simulink model "Laboratorio_5_SC2_Simulink_P3"  (R2019a)
settings: Solver=VariableStepAuto  StartTime=0.0  StopTime=1.5  RelTol=1e-3
values from neighbouring files (symbols this model uses):
  A_p3 = double(A_p3)    [Laboratorio_5_SC2.m]
  B_p3 = double(B_p3)    [Laboratorio_5_SC2.m]
  C1 = [1 0 0 0 ... (first row only)    [Laboratorio_5_SC2.m]
  C2 = eye(4)    [Laboratorio_5_SC2.m]
  D1 = [0; 0]    [Laboratorio_5_SC2.m]
  D2 = [0; 0; 0; 0]    [Laboratorio_5_SC2.m]
  F = 500e3    (= 500000)    [Laboratorio_5_SC2.m]
  fs_new = 20000    [Laboratorio_5_SC2.m]
  fv = 15020    [Laboratorio_5_SC2.m]
  init_con = [0; 1; 0; 0]    [Laboratorio_5_SC2.m]
libraries: fl_lib x13, nesl_utility x6
settings Model: Creator=Hector  LastModifiedBy=Hector

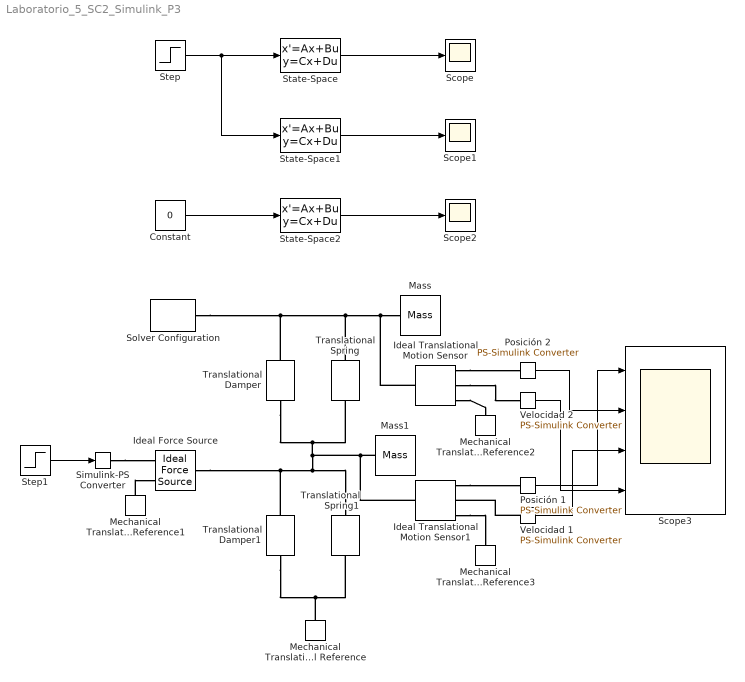
== system Laboratorio_5_SC2_Simulink_P3 ==
  Constant : Constant  Value=0
  Ideal Force Source : fl_lib/Mechanical/Mechanical Sources/Ideal Force Source
  Ideal Translational Motion Sensor : fl_lib/Mechanical/Mechanical Sensors/Ideal Translational Motion Sensor  offset=0 m
  Ideal Translational Motion Sensor1 : fl_lib/Mechanical/Mechanical Sensors/Ideal Translational Motion Sensor  offset=0 m
  Mass : fl_lib/Mechanical/Translational Elements/Mass  mass=M2 kg  v_specify=off  v_priority=High  v=0 m/s  v_nominal_specify=off  v_nominal_unit=m/s  v_nominal_value=1  f_specify=off  f_priority=None  f=0 N  f_nominal_specify=off  f_nominal_unit=N  f_nominal_value=1
  Mass1 : fl_lib/Mechanical/Translational Elements/Mass  mass=M1 kg  v_specify=off  v_priority=High  v=0 m/s  v_nominal_specify=off  v_nominal_unit=m/s  v_nominal_value=1  f_specify=off  f_priority=None  f=0 N  f_nominal_specify=off  f_nominal_unit=N  f_nominal_value=1
  Mechanical Translational Reference{,1..3} (4 alike) : fl_lib/Mechanical/Translational Elements/Mechanical Translational Reference
  Posición 1 : nesl_utility/PS-Simulink Converter  PhysicalDomain=network_engine_domain  SubClassName=ps_output  LeftPortType=input  RightPortType=output  PseudoPeriodic=off  Frequencies=[]  Unit=1  AffineConversion=off
  Posición 2 : nesl_utility/PS-Simulink Converter  PhysicalDomain=network_engine_domain  SubClassName=ps_output  LeftPortType=input  RightPortType=output  PseudoPeriodic=off  Frequencies=[]  Unit=1  AffineConversion=off
  Scope : Scope
  Scope1 : Scope
  Scope2 : Scope
  Scope3 : Scope  NumInputPorts=4
  Simulink-PS Converter : nesl_utility/Simulink-PS Converter  PhysicalDomain=network_engine_domain  SubClassName=ps_input  LeftPortType=input  RightPortType=output  PseudoPeriodic=off  Frequencies=[]  NoiseDistribution=none  NoiseParameters=[]  Unit=1  AffineConversion=off  FilteringAndDerivatives=provide  SimscapeFilterOrder=1  InputFilterTimeConstant=0.001  UdotUserProvided=0
  Solver Configuration : nesl_utility/Solver Configuration  PhysicalDomain=network_engine_domain  SubClassName=solver  LeftPortType=input  RightPortType=generic  Tones=[]  Harmonics=[]  SimulateNoise=off  Profile=off  UseLocalSampling=off  EnableSwitchedLinearOptims=on  FrequencyDomain=off  UseCCode=off  RelTol=0.001  AbsTol=1e-06  MinStep=1e-09  ToWorkspace=off  RevertToSquareIcSolve=off  NumHomotopyIterations=100  PhasorMode=off  PhasorModeNumHarmonics=1  DoDC=off  ResidualTolerance=1e-09  UseLocalSolver=off  LocalSolverChoice=NE_BACKWARD_EULER_ADVANCER  LocalSolverSampleTime=0.001  DoFixedCost=off  MaxNonlinIter=3  MaxModeIter=2  LinearAlgebra=auto  EquationFormulation=NE_TIME_EF  DelaysMemoryBudget=1024  AutomaticFiltering=on  FilteringTimeConstant=0.001  PartitionStorageMethod=AS_NEEDED  PartitionMemoryBudget=1024  PartitionMethod=ROBUST
  State-Space : StateSpace  A=A_p3  B=B_p3  C=C1  D=D1  InitialCondition=0
  State-Space1 : StateSpace  A=A_p3  B=B_p3  C=C2  D=D2  InitialCondition=0
  State-Space2 : StateSpace  A=A_p3  B=B_p3  C=C2  D=D2  InitialCondition=init_con
  Step : Step  Time=0  After=F  SampleTime=0
  Step1 : Step  Time=0  After=F  SampleTime=0
  Translational Damper : fl_lib/Mechanical/Translational Elements/Translational Damper  D=fs_new N/(m/s)  v_specify=off  v_priority=None  v=0 m/s  v_nominal_specify=off  v_nominal_unit=m/s  v_nominal_value=1  f_specify=off  f_priority=None  f=0 N  f_nominal_specify=off  f_nominal_unit=N  f_nominal_value=1
  Translational Damper1 : fl_lib/Mechanical/Translational Elements/Translational Damper  D=fv N/(m/s)  v_specify=off  v_priority=None  v=0 m/s  v_nominal_specify=off  v_nominal_unit=m/s  v_nominal_value=1  f_specify=off  f_priority=None  f=0 N  f_nominal_specify=off  f_nominal_unit=N  f_nominal_value=1
  Translational Spring : fl_lib/Mechanical/Translational Elements/Translational Spring  spr_rate=ks_new N/m  v_specify=off  v_priority=None  v=0 m/s  v_nominal_specify=off  v_nominal_unit=m/s  v_nominal_value=1  f_specify=off  f_priority=None  f=0 N  f_nominal_specify=off  f_nominal_unit=N  f_nominal_value=1  x_specify=off  x_priority=High  x=0 m  x_nominal_specify=off  x_nominal_unit=m  x_nominal_value=1
  Translational Spring1 : fl_lib/Mechanical/Translational Elements/Translational Spring  spr_rate=k N/m  v_specify=off  v_priority=None  v=0 m/s  v_nominal_specify=off  v_nominal_unit=m/s  v_nominal_value=1  f_specify=off  f_priority=None  f=0 N  f_nominal_specify=off  f_nominal_unit=N  f_nominal_value=1  x_specify=off  x_priority=High  x=0 m  x_nominal_specify=off  x_nominal_unit=m  x_nominal_value=1
  Velocidad 1 : nesl_utility/PS-Simulink Converter  PhysicalDomain=network_engine_domain  SubClassName=ps_output  LeftPortType=input  RightPortType=output  PseudoPeriodic=off  Frequencies=[]  Unit=1  AffineConversion=off
  Velocidad 2 : nesl_utility/PS-Simulink Converter  PhysicalDomain=network_engine_domain  SubClassName=ps_output  LeftPortType=input  RightPortType=output  PseudoPeriodic=off  Frequencies=[]  Unit=1  AffineConversion=off
  wires:
  Step1/1 -> Simulink-PS Converter/1
  Posición 2/1 -> Scope3/2
  Velocidad 2/1 -> Scope3/4
  Velocidad 1/1 -> Scope3/3
  Step/1 -> State-Space1/1, State-Space/1
  Constant/1 -> State-Space2/1
  Posición 1/1 -> Scope3/1
  State-Space2/1 -> Scope2/1
  State-Space/1 -> Scope/1
  State-Space1/1 -> Scope1/1
  connections:
  Solver Configuration/RConn1 -- Translational Damper/LConn1 -- Translational Spring/LConn1 -- Mass/LConn1 -- Ideal Translational Motion Sensor/LConn1
  Translational Spring/RConn1 -- Translational Damper/RConn1 -- Ideal Translational Motion Sensor1/LConn1 -- Mass1/LConn1 -- Translational Damper1/LConn1 -- Ideal Force Source/LConn1 -- Translational Spring1/LConn1
  Translational Spring1/RConn1 -- Translational Damper1/RConn1 -- Mechanical Translational Reference/LConn1
  Ideal Translational Motion Sensor1/RConn3 -- Posición 1/LConn1
  Ideal Translational Motion Sensor/RConn3 -- Posición 2/LConn1
  Mechanical Translational Reference1/LConn1 -- Ideal Force Source/RConn2
  Ideal Translational Motion Sensor/RConn1 -- Mechanical Translational Reference2/LConn1
  Ideal Translational Motion Sensor1/RConn1 -- Mechanical Translational Reference3/LConn1
  Velocidad 1/LConn1 -- Ideal Translational Motion Sensor1/RConn2
  Ideal Translational Motion Sensor/RConn2 -- Velocidad 2/LConn1
  Simulink-PS Converter/RConn1 -- Ideal Force Source/RConn1
